simulink model "Citation"  (R2018a)
settings: Solver=ode5  StartTime=0.0  StopTime=500  FixedStep=0.01  RelTol=1e-3  EnableMultiTasking=on
InitFcn:
  | initcit
values from neighbouring files (symbols this model uses):
  aeroinit = [dp_ini;inicoef('CX0');inicoef('CXa');inicoef('CXa2');inicoef('CXq')     ;inicoef('CXde');inicoef('CY0');inicoef('CYB');inicoef('CYp');inicoef('CYr')     ;inicoef('CYda');inicoef('CYdr');inicoef('CZ0');inicoef('CZa');inicoef('CZq')     ;inicoef('CZde');inicoef('Cl0');inicoef('ClB');inicoef('Clp');inicoef('Clr')     ;inicoef('Clda');inicoef('Cldr');inicoef('Cm0');inicoef('Cma');inicoef('Cmq')     ; ...(+113 chars)    [initcit.m]
  h_l_old = zeros(6,sample_size)    [initcit.m]
  h_m_old = zeros(4,sample_size)    [initcit.m]
  h_n_old = zeros(6,sample_size)    [initcit.m]
  h_X_old = zeros(5,sample_size)    [initcit.m]
  h_Y_old = zeros(6,sample_size)    [initcit.m]
  h_Z_old = zeros(4,sample_size)    [initcit.m]
  I = [massinit(5),0, -massinit(8);0, massinit(6),0;-massinit(8),0, massinit(7)]    [initcit.m]
  p_l = [inicoef('Cl0');inicoef('ClB');inicoef('Clp');inicoef('Clr')     ;inicoef('Clda');inicoef('Cldr')].*ones(6,sample_size)    [initcit.m]
  p_m = [inicoef('Cm0');inicoef('Cma');inicoef('Cmq')     ;inicoef('Cmde')].*ones(4,sample_size)    [initcit.m]
  p_n = 0.71*ones(6,sample_size)    [initcit.m]
  p_X = [inicoef('CX0');inicoef('CXa');inicoef('CXa2');inicoef('CXq')     ;inicoef('CXde')].*ones(5,sample_size)    [initcit.m]
  p_Y = [inicoef('CY0');inicoef('CYB');inicoef('CYp');inicoef('CYr')     ;inicoef('CYda');inicoef('CYdr')].*ones(6,sample_size)    [initcit.m]
  p_Z = [inicoef('CZ0');inicoef('CZa');inicoef('CZq')     ;inicoef('CZde')].*ones(4,sample_size)    [initcit.m]
  Pcov_l = 10000*eye(6)    [initcit.m]
  Pcov_m = 10000*eye(4)    [initcit.m]
  Pcov_n = 10000*eye(6)    [initcit.m]
  Pcov_X = 10000*eye(5)    [initcit.m]
  Pcov_Y = 10000*eye(6)    [initcit.m]
  Pcov_Z = 10000*eye(4)    [initcit.m]
  T0 = 288.15    [rho_test.m]
  Vw915 = 0    [initcit.m]
  winddir = 45*(pi/180)    (= 0.785398163397)    [initcit.m]
  x0 = []    [cessnac550_3d_sfnc.m]    (also in sfunxyauto.m)
  y_l = zeros(1,sample_size)    [initcit.m]
  y_l_est_old = zeros(size(y_l))    [initcit.m]
  y_m = zeros(1,sample_size)    [initcit.m]
  y_m_est_old = zeros(size(y_m))    [initcit.m]
  y_n = zeros(1,sample_size)    [initcit.m]
  y_n_est_old = zeros(size(y_n))    [initcit.m]
  y_X = zeros(1,sample_size)    [initcit.m]
  y_X_est_old = zeros(size(y_X))    [initcit.m]
  y_Y = zeros(1,sample_size)    [initcit.m]
  y_Y_est_old = zeros(size(y_Y))    [initcit.m]
  y_Z = zeros(1,sample_size)    [initcit.m]
  y_Z_est_old = zeros(size(y_Z))    [initcit.m]
undefined symbols (not defined in the file or in its folder): chord, cv1, cv2, cv3, cv4, deltagmax1, deltagmax2, deltagmax3, deltagmax4, Deng, ealphag, ealphas, g0, hDME, hGS, kt1, kt2, kt3, lh, massinit, matbuaf, matdaf, matdam, matdbbf, matdeaf, matdgaf, matdqaf, matduaf, matdwaw, matedhr, mateif, matelhr, matemhr, matemv1, matemv2, matemve, matetam, mateuaf, matfaaf, matfaxl, matff, matibaf, matibb, matibmh, matipaf, matipmh, matiraf, matiuaf, matiwaf, matlaf, matlam, matleaf, matleam, matlgaf, matlqaf, matluaf, matmaaf, matmaam, matmaf, matmam ... (+75)
libraries: simulink x5, templibrary x3, vrlib x1
(part 1 of 6)
settings Model: ExtModeTrigMode=oneshot  ExtModeArmWhenConnect=off  Creator=laurensvaneykeren  LastModifiedBy=jelle
settings DataIOCC: SaveFormat=Array  SignalLoggingName=sigsOut
settings OptimizationCC: BooleanDataType=off  ExpressionDepthLimit=2147483647  LifeSpan=inf
settings DebuggingCC: SaveWithParameterizedLinksMsg=none  UnderspecifiedInitializationDetection=Classic  MergeDetectMultiDrivingBlocksExec=none  SignalResolutionControl=TryResolveAllWithWarning  MultiTaskDSMMsg=warning  MultiTaskCondExecSysMsg=none  FcnCallInpInsideContextMsg=warning  StateNameClashWarn=warning  SFUnexpectedBacktrackingDiag=warning  SFNoUnconditionalDefaultTransitionDiag=warning  SFExecutionAtInitializationDiag=none
settings HardwareCC: ProdBitPerPointer=32  ProdBitPerSizeT=32  ProdBitPerPtrDiffT=32  ProdLargestAtomicFloat=None  ProdIntDivRoundTo=Undefined  ProdEndianess=Unspecified  ProdWordSize=32  ProdHWDeviceType=32-bit Generic  TargetUnknown=on
settings ModelReferenceCC: PropagateSignalLabelsOutOfModel=off
settings RTWCC: SystemTargetFile=grt_malloc.tlc  GenCodeOnly=on  TemplateMakefile=grt_malloc_default_tmf
settings CodeAppCC: StateflowObjectComments=on
settings GRTTargetCC: TargetLangStandard=C89/C90 (ANSI)  CombineOutputUpdateFcns=off  GRTInterface=on  UseMalloc=on
settings ConfigComp: CovMetricSettings=dw  CovHtmlReporting=on  CovSaveCumulativeToWorkspaceVar=on  CovSaveSingleToWorkspaceVar=on  CovExternalEMLEnable=off

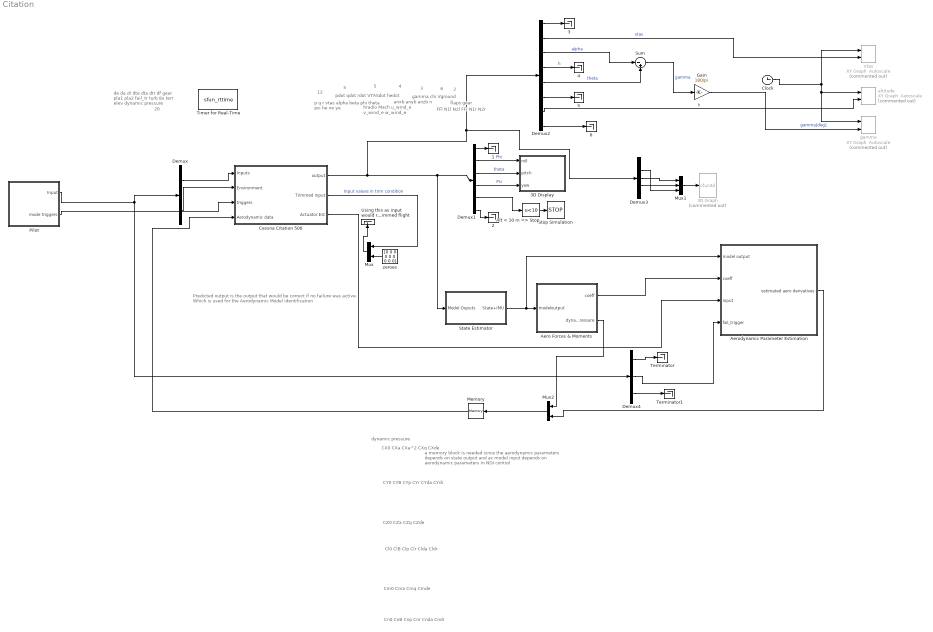
== system Citation ==
  note: a memory block is needed since the aerodynamic parameters depends on state output and ac model input depends on aerodynamic parameters in NDI control
  note: Predicted output is the output that would be correct if no failure was active.
      | Which is used for the Aerodynamic Model identification
  note: de
      | da
      | dr
      | dte
      | dta
      | dtr
      | df
      | gear
      | pla1
      | pla2
      | fail_tr
      | turb 8x
      | terr elev
      | dynamic pressure
  note: p
      | q
      | r
      | vtas
      | alpha
      | beta
      | phi
      | theta
      | psi
      | he
      | xe
      | ye
  note: pdot
      | qdot
      | rdot
      | VTASdot
      | hedot
  note: hradio
      | Mach
      | u_wind_e
      | v_wind_e
      | w_wind_e
  note: anxb
      | anyb
      | anzb
      | n
  note: gamma
      | chi
      | Vground
  note: flaps
      | gear
  note: FFl
      | N1l
      | N2l
      | FFr
      | N1r
      | N2r
  note: 12
  note: 5
  note: 5
  note: 4
  note: 3
  note: 6
  note: 2
  note: 20
  note: Cn0
      | CnB
      | Cnp
      | Cnr
      | Cnda
      | Cndr
  note: CZ0
      | CZa
      | CZq
      | CZde
  note: Cm0
      | Cma
      | Cmq
      | Cmde
  note: CY0
      | CYB
      | CYp
      | CYr
      | CYda
      | CYdr
  note: Cl0
      | ClB
      | Clp
      | Clr
      | Clda
      | Cldr
  note: CX0
      | CXa
      | CXa^2
      | CXq
      | CXde
  note: dynamic pressure
  {1..6} (6 alike) : Terminator
  3D Display : Subsystem
  3D Graph : S-Function  Commented=on  LoadFcn=if exist('sfun3d','file'), sfun3d([],[],[],'LoadBlock'); end  FunctionName=sfun3d  Parameters=ax,T,np,cp,gd,ls,mk,mx,hd,tb  SFunctionDeploymentMode=off  EnableBusSupport=off  mask(3D Graph){np=1, ax=[-5000 5000 -5000 5000 0 10000], mx=1e8, T=0.01, cp=[1 1 0.5], gd=on, hd=on, tb=on, ls=-, mk=none}
      mask prompts: np "Number of moving points (lines)"; ax "Range: [xmin xmax  ymin ymax zmin zmax]"; mx "Max number of points in each line"; T "Sampling Time"; cp "Camera position (use [0 0 1] for 2D XY view)"; gd "Grid (on|off)"; hd "HeadMarkers (on|off)"; tb "Toolbar (on|off)"; ls "LineStyle"; mk "LineMarker"
      mask help:
      | This block plots the position of several points in the XYZ space. The input contains the coordinates of all the points (x1,y1,z1,x2,y2,z2,...).
      | The number of moving points (lines), the XYZ ranges, sampling time, camera position, and grid (among other things) can be set as mask parameters.
      settings: CopyFcn=if exist('sfun3d','file'), sfun3d([],[],[],'CopyBlock'); end  DeleteFcn=if exist('sfun3d','file'), sfun3d([],[],[],'DeleteBlock'); end  NameChangeFcn=if exist('sfun3d','file'), sfun3d([],[],[],'NameChange'); end
      mask Help:
      | This block plots the position of several points in the XYZ space. The input contains the coordinates of all the points (x1,y1,z1,x2,y2,z2,...).
      | The number of moving points (lines), the XYZ ranges, sampling time, camera position, and grid (among other things) can be set as mask parameters.
      mask TypeOptions ls: - | -- | : | -. | none
      mask TypeOptions mk: none | . | + | o | * | x | square | diamond | v | ^ | > | < | pentagram | hexagram
      mask Display: plot([.05 .95 .95 .05 .05],[.45 .45 .95 .95 .45], 0.5+cos(0:0.1:2*pi)*0.3,0.7+sin(0:0.1:2*pi)*0.2)
  "Aero Forces & Moments " : Subsystem
  Aerodynamic Parameter Estimation : Subsystem
  Alt < 10 m => Stop : Fcn  Expr=u<10
  Cessna Citation 500 : Subsystem  mask(Citation Aircraft Model){trimdatafile=example.tri}
      mask prompts: trimdatafile "Trim Condition"
      mask init:
      | initcit;
      mask Display:
      | image(imread('Citation.jpg'))
      | port_label('input', 1, 'Inputs')
      | port_label('input', 2, 'Environment')
      | port_label('input', 4, 'Aerodynamic Data')
      | port_label('input', 3, 'Mode Triggers')
      | port_label('output', 1, 'Outputs')
      | port_label('output', 2, 'Trim inputs')
      | port_label('output', 3, 'Predicted Output')
  Clock : Clock
  Demux : Demux  Outputs=[11 9]
  Demux1 : Demux  Outputs=[6 1 1 1 1 27]
  Demux2 : Demux  Outputs=[3 1 1 2 1 1 1 27]
  Demux3 : Demux  Outputs=[9 1 1 1 25]
  Demux4 : Demux  Outputs=[10 1 9]
  Gain : Gain  Gain=180/pi
  Memory : Memory  InitialCondition=aeroinit
  Mux : Mux  Inputs=2
  Mux1 : Mux  Inputs=3
  Mux2 : Mux  Inputs=2
  Pilot : Subsystem
  "State Estimator " : Subsystem
  Stop Simulation : Stop
  Sum : Sum  Inputs=|-+
  Terminator : Terminator
  Terminator1 : Terminator
  Timer for Real-Time : S-Function  FunctionName=sfun_rttime  Parameters=1  SFunctionDeploymentMode=off  EnableBusSupport=off
  Using this as input would result in trimmed flight : Terminator
  Vtas : templibrary/XY Graph  Autoscale  Commented=on  xmin=-1  xmax=1  ymin=-1  ymax=1  st=0
  altitude : templibrary/XY Graph  Autoscale  Commented=on  xmin=-1  xmax=1  ymin=-1  ymax=1  st=0
      link override S-Function: Parameters="[xmin xmax ymin ymax],  st"
  gamma : templibrary/XY Graph  Autoscale  Commented=on  xmin=-1  xmax=1  ymin=-1  ymax=1  st=0
  zeroes : Constant  Value=[0 0 0 0 0 0 0 0 0]
  wires:
  Demux/1 -> Cessna Citation 500/1(Inputs)
  Pilot/1(Input) -> Demux/1, Demux4/1
  Cessna Citation 500/1(output) -> Demux3/1, Demux2/1, "State Estimator "/1(Model Ouputs), Demux1/1
  Demux/2 -> Cessna Citation 500/2(Environment)
  Cessna Citation 500/2(Trimmed input) -> Mux/1  "Input values in trim condition"
  zeroes/1 -> Mux/2
  Mux/1 -> Using this as input would result in trimmed flight/1
  Demux1/1 -> 1/1
  Demux1/5 -> Alt < 10 m => Stop/1
  Demux1/2 -> 3D Display/1(roll)  "Phi"
  Demux1/3 -> 3D Display/2(pitch)  "theta"
  Demux1/4 -> 3D Display/3(yaw)  "Psi"
  Alt < 10 m => Stop/1 -> Stop Simulation/1
  Demux1/6 -> 2/1
  "State Estimator "/1(State+IMU) -> Aerodynamic Parameter Estimation/1("model output "), "Aero Forces & Moments "/1(modeloutput)
  Cessna Citation 500/3(Actuator Est) -> Aerodynamic Parameter Estimation/3("input ")
  "Aero Forces & Moments "/1(coeff) -> Aerodynamic Parameter Estimation/2("coeff ")
  Demux2/1 -> 3/1
  Demux2/2 -> Vtas/2  "vtas"
  Demux2/3 -> Sum/1  "alpha"
  Demux2/4 -> 4/1  "h"
  Demux2/5 -> Sum/2  "theta"
  Demux2/7 -> altitude/2  "h"
  Demux2/6 -> 5/1
  Demux2/8 -> 6/1
  Sum/1 -> Gain/1  "gamma"
  Gain/1 -> gamma/2  "gamma[deg]"
  Demux3/2 -> Mux1/3
  Demux3/3 -> Mux1/1
  Demux3/4 -> Mux1/2
  Mux1/1 -> 3D Graph/1
  Clock/1 -> gamma/1, altitude/1, Vtas/1
  Demux4/2 -> Aerodynamic Parameter Estimation/4("fail_trigger ")
  Demux4/1 -> Terminator/1
  Demux4/3 -> Terminator1/1
  Aerodynamic Parameter Estimation/1(estimated aero derivatives) -> Mux2/2
  "Aero Forces & Moments "/2("dynamic pressure ") -> Mux2/1
  Mux2/1 -> Memory/1
  Memory/1 -> Cessna Citation 500/4("Aerodynamic data ")
  Pilot/2("mode triggers ") -> Cessna Citation 500/3(triggers)

== system Citation/3D Display ==
  roll : Inport
  pitch : Inport  Port=2
  yaw : Inport  Port=3
  Mux1 : Mux
  Position : Subsystem
  S-Function : S-Function  FunctionName=cessnac550_3d_sfnc  SFunctionDeploymentMode=off  EnableBusSupport=off
  Stop Simulation : Stop
  wires:
  roll/1 -> Mux1/1
  Position/1(Out1) -> Mux1/4
  pitch/1 -> Mux1/2
  yaw/1 -> Mux1/3
  Mux1/1 -> S-Function/1
  S-Function/1 -> Stop Simulation/1

== system Citation/Aero Forces & Moments  ==
  note: Kinematic Force Coeffient determination
  note: anxb
      | anyb
      | anzb
      | n
  note: hradio
      | Mach
      | u_wind_e
      | v_wind_e
      | w_wind_e
  note: p
      | q
      | r
      | vtas
      | alpha
      | beta
      | phi
      | theta
      | psi
      | he
      | xe
      | ye
  note: gamma
      | chi
      | Vground
  note: pdot
      | qdot
      | rdot
      | VTASdot
      | hedot
  note: FFl
      | N1l
      | N2l
      | FFr
      | N1r
      | N2r
  note: flaps
      | gear
  note: 6
  note: 5
  note: 12
  note: 3
  note: 5
  note: 4
  note: 2
  note: CX
      | CY
      | CZ
      | Cl
      | Cm
      | Cn
  modeloutput : Inport
  Aerodynamic Force Components : Subsystem
  Aerodynamic Moment Components : Subsystem
  Calculate Dynamic Pressure : Subsystem
  Mux : Mux  Inputs=2
  coeff : Outport
  "dynamic pressure " : Outport  Port=2
  wires:
  Aerodynamic Force Components/1(Out1) -> Mux/1
  modeloutput/1 -> Calculate Dynamic Pressure/1(In1), Aerodynamic Moment Components/1("State "), Aerodynamic Force Components/1("model output ")
  Calculate Dynamic Pressure/1(Out1) -> "dynamic pressure "/1, Aerodynamic Moment Components/2("Dynamic Pressure "), Aerodynamic Force Components/2(dynamic pressure)
  Aerodynamic Moment Components/1(Out1) -> Mux/2
  Mux/1 -> coeff/1

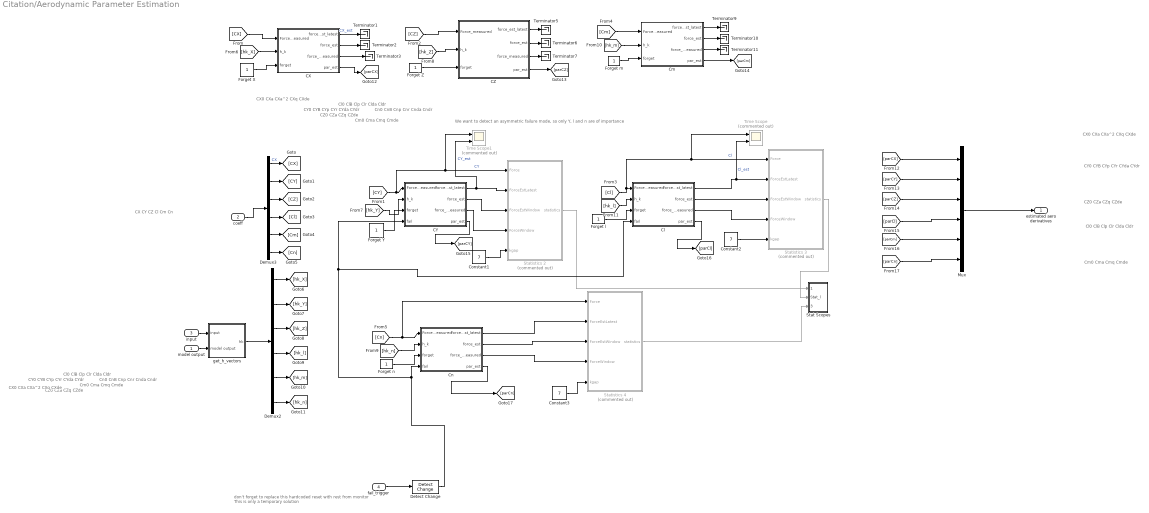
== system Citation/Aerodynamic Parameter Estimation ==
  note: don't forget to replace this hardcoded reset with rest from monitor
      | This is only a temporary solution
  note: We want to detect an asymmetric failure mode, so only Y, l and n are of importance
  note: CX
      | CY
      | CZ
      | Cl
      | Cm
      | Cn
  note: CX0
      | CXa
      | CXa^2
      | CXq
      | CXde
  note: CY0
      | CYB
      | CYp
      | CYr
      | CYda
      | CYdr
  note: CZ0
      | CZa
      | CZq
      | CZde
  note: Cl0
      | ClB
      | Clp
      | Clr
      | Clda
      | Cldr
  note: Cm0
      | Cma
      | Cmq
      | Cmde
  note: Cn0
      | CnB
      | Cnp
      | Cnr
      | Cnda
      | Cndr
  note: Cm0
      | Cma
      | Cmq
      | Cmde
  note: Cn0
      | CnB
      | Cnp
      | Cnr
      | Cnda
      | Cndr
  note: CY0
      | CYB
      | CYp
      | CYr
      | CYda
      | CYdr
  note: CZ0
      | CZa
      | CZq
      | CZde
  note: CX0
      | CXa
      | CXa^2
      | CXq
      | CXde
  note: Cl0
      | ClB
      | Clp
      | Clr
      | Clda
      | Cldr
  note: Cl0
      | ClB
      | Clp
      | Clr
      | Clda
      | Cldr
  note: CY0
      | CYB
      | CYp
      | CYr
      | CYda
      | CYdr
  note: Cm0
      | Cma
      | Cmq
      | Cmde
  note: CX0
      | CXa
      | CXa^2
      | CXq
      | CXde
  note: CZ0
      | CZa
      | CZq
      | CZde
  "model output " : Inport
  "coeff " : Inport  Port=2
  "input " : Inport  Port=3
  "fail_trigger " : Inport  Port=4
  CX : Subsystem
  CY : Subsystem
  CZ : Subsystem
  Cl : Subsystem
  Cm : Subsystem
  Cn : Subsystem
  Constant1 : Constant  Value=7
  Constant2 : Constant  Value=7
  Constant3 : Constant  Value=7
  Demux2 : Demux  Outputs=[5 6 4 6 4 6]
  Demux3 : Demux  Outputs=[1 1 1 1 1 1]
  Detect Change : simulink/Logic and Bit Operations/Detect Change  vinit=0  OutDataTypeStr=boolean
  Forget X : Constant
  Forget Y : Constant
  Forget Z : Constant
  Forget l : Constant
  Forget m : Constant
  Forget n : Constant
  Mux : Mux  Inputs=6
  "Stat Scopes " : Subsystem
  Statistics 2 : Subsystem  Commented=on
  Statistics 3 : Subsystem  Commented=on
  Statistics 4 : Subsystem  Commented=on
  Terminator{1..3,5..7,9..11} (9 alike) : Terminator
  Time Scope : Scope  Commented=on  NumInputPorts=2
  Time Scope1 : Scope  Commented=on  NumInputPorts=2
  get_h_vectors : Subsystem
  estimated aero derivatives : Outport
  wires:
  "input "/1 -> get_h_vectors/1(input)
  "model output "/1 -> get_h_vectors/2(model output)
  get_h_vectors/1(hk) -> Demux2/1
  "coeff "/1 -> Demux3/1
  Demux3/2 -> [CY]
  CX/4(par_est) -> [parCX]
  Forget X/1 -> CX/3(forget)
  Forget Y/1 -> CY/3(forget)
  Forget Z/1 -> CZ/3(forget)
  Forget l/1 -> Cl/3(forget)
  Forget m/1 -> Cm/3(forget)
  Forget n/1 -> Cn/3(forget)
  CY/1(force_est_latest) -> Time Scope1/2, Statistics 2/2(ForceEstLatest)  "CY_est"
  CY/2(force_est) -> Statistics 2/3(ForceEstWindow)
  CY/3(force_measured) -> Statistics 2/4(ForceWindow)
  Constant1/1 -> Statistics 2/5("kgap ")
  Cl/1(force_est_latest) -> Time Scope/2, Statistics 3/2(ForceEstLatest)  "Cl_est"
  Cl/2(force_est) -> Statistics 3/3(ForceEstWindow)
  Cl/3(force_measured) -> Statistics 3/4(ForceWindow)
  Constant2/1 -> Statistics 3/5("kgap ")
  Cn/1(force_est_latest) -> Statistics 4/2(ForceEstLatest)
  Cn/2(force_est) -> Statistics 4/3(ForceEstWindow)
  Constant3/1 -> Statistics 4/5("kgap ")
  Demux3/1 -> [CX]  "CX"
  [CX] -> CX/1(Force_measured)
  [CY] -> Time Scope1/1, Statistics 2/1(Force), CY/1(Force_measured)  "CY"
  Demux3/3 -> [CZ]
  [CZ] -> CZ/1(Force_measured)
  Demux3/4 -> [Cl]
  [Cl] -> Time Scope/1, Statistics 3/1(Force), Cl/1(Force_measured)  "Cl"
  Demux3/5 -> [Cm]
  [Cm] -> Cm/1(Force_measured)
  Demux3/6 -> [Cn]
  [Cn] -> Statistics 4/1(Force), Cn/1(Force_measured)
  Demux2/1 -> [hk_X]
  Demux2/2 -> [hk_Y]
  Demux2/3 -> [hk_Z]
  Demux2/4 -> [hk_l]
  Demux2/5 -> [hk_m]
  Demux2/6 -> [hk_n]
  [hk_X] -> CX/2(h_k)
  [hk_Y] -> CY/2(h_k)
  [hk_Z] -> CZ/2(h_k)
  [hk_l] -> Cl/2(h_k)
  [hk_m] -> Cm/2(h_k)
  [hk_n] -> Cn/2(h_k)
  Cn/3(force_measured) -> Statistics 4/4(ForceWindow)
  CX/1(force_est_latest) -> Terminator1/1  "CX_est"
  CX/2(force_est) -> Terminator2/1
  CX/3(force_measured) -> Terminator3/1
  CY/4(par_est) -> [parCY]
  CZ/2(force_est) -> Terminator6/1
  CZ/3(force_measured) -> Terminator7/1
  CZ/1(force_est_latest) -> Terminator5/1
  Cm/1(force_est_latest) -> Terminator9/1
  Cm/2(force_est) -> Terminator10/1
  Cm/3(force_measured) -> Terminator11/1
  Cm/4(par_est) -> [parCm]
  Statistics 4/1(statistics) -> "Stat Scopes "/3(Stat_n)
  Statistics 3/1(statistics) -> "Stat Scopes "/2(Stat_l)
  Statistics 2/1(statistics) -> "Stat Scopes "/1(Stat_Y)
  "fail_trigger "/1 -> Detect Change/1
  Detect Change/1 -> Cl/4("fail "), CY/4(fail), Cn/4("fail ")
  CZ/4(par_est) -> [parCZ]
  Cl/4(par_est) -> [parCl]
  Cn/4(par_est) -> [parCn]
  [parCX] -> Mux/1
  [parCY] -> Mux/2
  [parCZ] -> Mux/3
  [parCl] -> Mux/4
  [parCm] -> Mux/5
  [parCn] -> Mux/6
  Mux/1 -> estimated aero derivatives/1

== system Citation/Cessna Citation 500 ==
  note: output is actuator deflection before failure
  note: p
      | q
      | r
      | vtas
      | alpha
      | beta
      | phi
      | theta
      | psi
      | he
      | xe
      | ye
  note: de
      | da
      | dr
      | dte
      | dta
      | dtr
      | df
      | gear
      | pla1
      | pla2
  note: pdot
      | qdot
      | rdot
      | VTASdot
      | hedot
  note: hradio
      | Mach
      | u_wind_e
      | v_wind_e
      | w_wind_e
  note: anxb
      | anyb
      | anzb
      | n
  note: gamma
      | chi
      | Vground
  note: turb 8x
      | terr_elev
  note: flaps
      | gear
  note: de
      | da
      | dr
      | dte
      | dta
      | dtr
      | df
      | gear
      | pla1
      | pla2
  note: FFl
      | N1l
      | N2l
      | FFr
      | N1r
      | N2r
  note: fail_aileron
  Inputs : Inport
  Environment : Inport  Port=2
  triggers : Inport  Port=3
  "Aerodynamic data " : Inport  Port=4
  Actuators : Subsystem
  Citation model DASMAT : Subsystem
  Controllers : Subsystem
  Demux : Demux  Outputs=[10 1]
  Demux4 : Demux  Outputs=[8 2]
  Mux1 : Mux  Inputs=7
  Mux2 : Mux  Inputs=2
  trim conditions : Subsystem
  ua sel : Selector  IndexOptions=Index vector (dialog)  Indices=[5 6]  OutputSizes=1
  xdot sel : Selector  IndexOptions=Index vector (dialog)  Indices=[1 2 3 4 10]  OutputSizes=1
  yacc sel : Selector  IndexOptions=Index vector (dialog)  Indices=[4 5 6 15]  OutputSizes=1
  yair sel : Selector  IndexOptions=Index vector (dialog)  Indices=[6 9 22 23 24]  OutputSizes=1
  yfp sel : Selector  IndexOptions=Index vector (dialog)  Indices=[1 2 15]  OutputSizes=1
  ypp sel : Selector  IndexOptions=Index vector (dialog)  Indices=[2 3 4 13 14 15]  OutputSizes=1
  output : Outport
  Trimmed input : Outport  Port=2
  Actuator Est : Outport  Port=3
  wires:
  Mux1/1 -> output/1
  Citation model DASMAT/1(x) -> Mux1/1, Controllers/1(state)
  Demux4/1 -> Citation model DASMAT/1(ua), ua sel/1
  Demux4/2 -> Citation model DASMAT/2(ut)
  Citation model DASMAT/3(yair) -> yair sel/1
  yair sel/1 -> Mux1/3
  Citation model DASMAT/2(xdot) -> xdot sel/1
  xdot sel/1 -> Mux1/2
  yacc sel/1 -> Mux1/4
  Citation model DASMAT/4(yacc) -> yacc sel/1
  yfp sel/1 -> Mux1/5
  Citation model DASMAT/5(yfp) -> yfp sel/1
  Actuators/1(Actuator_True) -> Demux4/1
  trim conditions/1(ua) -> Mux2/1
  trim conditions/2(ut) -> Mux2/2
  Mux2/1 -> Trimmed input/1
  Controllers/1(control inputs) -> Actuators/1(In)
  ua sel/1 -> Mux1/7
  Citation model DASMAT/6(ypp) -> ypp sel/1
  ypp sel/1 -> Mux1/6
  Actuators/2(Actuator_est) -> Actuator Est/1
  Inputs/1 -> Demux/1
  Demux/1 -> Controllers/2(inputs)
  Demux/2 -> Actuators/2("failure trigger ")
  Environment/1 -> Citation model DASMAT/3(Environment)
  "Aerodynamic data "/1 -> Controllers/3(aerodata)
  triggers/1 -> Controllers/4("triggers ")

== system Citation/Pilot ==
  note: de
      | da
      | dr
      | dte
      | dta
      | dtr
      | df
      | gear
      | pla1
      | pla2
      | failure_tr
      | turb 8x
      | terr elev
  Joystick : Subsystem
  Mux : Mux  Inputs=13
  "button2toggle " : Subsystem
  button2toggle 1 : Subsystem
  da trim : Constant  Value=0
  de trim : Constant  Value=0
  delta flaps : Constant  Value=0
  dr trim : Constant  Value=0
  gear (ON=1/OFF=0) : Constant  Value=0
  terr elev : Constant  Value=0
  turb 8x : Constant  Value=zeros(1,8)
  Input : Outport
  "mode triggers " : Outport  Port=2
  wires:
  Mux/1 -> Input/1
  Joystick/1(delta elevator) -> Mux/1
  Joystick/3(delta rudder) -> Mux/3
  da trim/1 -> Mux/5
  de trim/1 -> Mux/4
  Joystick/2(delta aileron) -> Mux/2
  turb 8x/1 -> Mux/12
  terr elev/1 -> Mux/13
  Joystick/4(Throttle setting) -> Mux/10, Mux/9
  gear (ON=1/OFF=0)/1 -> Mux/8
  dr trim/1 -> Mux/6
  delta flaps/1 -> Mux/7
  Joystick/5("Failure Button ") -> "button2toggle "/1(In1)
  "button2toggle "/1(Out1) -> Mux/11
  Joystick/6(NDI Button) -> button2toggle 1/1(In1)
  button2toggle 1/1(Out1) -> "mode triggers "/1

== system Citation/State Estimator  ==
  note: It is assumed that the model ouputs are perfect measurements
  Model Ouputs : Inport
  State+IMU : Outport
  wires:
  Model Ouputs/1 -> State+IMU/1

== system Citation/3D Display/Position ==
  Mux2 : Mux  Inputs=3
  x : Constant  Value=0
  y : Constant  Value=0
  z : Constant  Value=0
  Out1 : Outport
  wires:
  y/1 -> Mux2/2
  z/1 -> Mux2/3
  x/1 -> Mux2/1
  Mux2/1 -> Out1/1

== system Citation/Aero Forces & Moments /Aerodynamic Force Components ==
  note: Massinit
      | [mass cg? ? ? Ixx Iyy Izz Ixz]
  note: State
  note: accelerations are given in [g]
  note: p
      | q
      | r
      | vtas
      | alpha
      | beta
      | phi
      | theta
      | psi
      | he
      | xe
      | ye
  note: gamma
      | chi
      | Vground
  note: hradio
      | Mach
      | u_wind_e
      | v_wind_e
      | w_wind_e
  note: anxb
      | anyb
      | anzb
      | n
  note: 5
  note: 12
  note: 4
  note: flaps
      | gear
  note: 3
  note: 6
  note: FFl
      | N1l
      | N2l
      | FFr
      | N1r
      | N2r
  note: 5
  note: pdot
      | qdot
      | rdot
      | VTASdot
      | hedot
  note: 2
  "model output " : Inport
  dynamic pressure : Inport  Port=2
  Constant : Constant  Value=massinit
  Demux : Demux  Outputs=[22 3 12]
  Demux2 : Demux  Outputs=[1 7]
  Divide : Product  Inputs=*/
  Gain : Gain  Gain=g0
  Product : Product
  Product2 : Product
  Terminator1 : Terminator
  Terminator2 : Terminator
  Terminator4 : Terminator
  Wing Area : Constant  Value=S
  Out1 : Outport
  wires:
  Demux/2 -> Gain/1
  Gain/1 -> Product2/1
  dynamic pressure/1 -> Product/1
  Wing Area/1 -> Product/2
  Product2/1 -> Divide/1
  Divide/1 -> Out1/1
  Product/1 -> Divide/2
  Demux/1 -> Terminator1/1
  Demux/3 -> Terminator2/1
  "model output "/1 -> Demux/1
  Demux2/1 -> Product2/2  "mass"
  Constant/1 -> Demux2/1
  Demux2/2 -> Terminator4/1

== system Citation/Aero Forces & Moments /Aerodynamic Moment Components ==
  note: p
      | q
      | r
      | vtas
      | alpha
      | beta
      | phi
      | theta
      | psi
      | he
      | xe
      | ye
  note: gamma
      | chi
      | Vground
  note: hradio
      | Mach
      | u_wind_e
      | v_wind_e
      | w_wind_e
  note: anxb
      | anyb
      | anzb
      | n
  note: 5
  note: 12
  note: 4
  note: flaps
      | gear
  note: 3
  note: 6
  note: FFl
      | N1l
      | N2l
      | FFr
      | N1r
      | N2r
  note: 5
  note: pdot
      | qdot
      | rdot
      | VTASdot
      | hedot
  note: 2
  note: Massinit
      | [mass cg? ? ? Ixx Iyy Izz Ixz]
  "State " : Inport
  "Dynamic Pressure " : Inport  Port=2
  Cl : Subsystem
  Cm : Subsystem
  Cn : Subsystem
  Mux : Mux  Inputs=3
  Out1 : Outport
  wires:
  "State "/1 -> Cl/1(model output), Cm/1("model output "), Cn/1(model output)
  "Dynamic Pressure "/1 -> Cn/2(Dynamic Pressure), Cm/2(Dynamic Pressure), Cl/2(Dynamic Pressure)
  Cl/1(Cl) -> Mux/1
  Cn/1(Cn) -> Mux/3
  Cm/1(Cm) -> Mux/2
  Mux/1 -> Out1/1

== system Citation/Aero Forces & Moments /Calculate Dynamic Pressure ==
  note: Dynamic Pressure
  In1 : Inport
  Calculate Air Density : MATLAB Function  TreatAsAtomicUnit=on
  Demux : Demux  Outputs=[3 1 33]
  Gain : Gain  Gain=0.5
  Product : Product
  Product1 : Product
  Terminator1 : Terminator
  Terminator2 : Terminator
  Out1 : Outport
  wires:
  Product/1 -> Product1/1  "V^2"
  Demux/3 -> Terminator2/1
  Demux/2 -> Product/2, Product/1  "Vtas"
  In1/1 -> Demux/1, Calculate Air Density/1(state)
  Product1/1 -> Gain/1
  Calculate Air Density/1(rho) -> Product1/2  "Rho"
  Demux/1 -> Terminator1/1
  Gain/1 -> Out1/1  "0.5*RHO*v^2"

== system Citation/Aerodynamic Parameter Estimation/CX ==
  note: counter is still obsolete
  note: if lambda=1 => no forgetting
  Force_measured : Inport
  h_k : Inport  Port=2
  forget : Inport  Port=3
  MATLAB Function : MATLAB Function  TreatAsAtomicUnit=on
  Memory1 : Memory
  Memory10 : Memory  InitialCondition=y_X
  Memory11 : Memory  InitialCondition=h_X_old
  Memory7 : Memory  InitialCondition=p_X
  Memory8 : Memory  InitialCondition=Pcov_X
  Memory9 : Memory  InitialCondition=y_X_est_old
  Selector : Selector  NumberOfDimensions=2  InputPortWidth=1  IndexOptions=Index vector (dialog),Index vector (dialog)  Indices=[1:5],1  OutputSizes=1,1
  Terminator : Terminator
  force_est_latest : Outport
  force_est : Outport  Port=2
  force_measured : Outport  Port=3
  par_est : Outport  Port=4
  wires:
  Memory9/1 -> MATLAB Function/6("y_est_old ")
  MATLAB Function/1(P_cov) -> Memory8/1
  Memory10/1 -> MATLAB Function/5("y_old ")
  MATLAB Function/5(h_old) -> Memory11/1
  Memory11/1 -> MATLAB Function/7("h_old ")
  MATLAB Function/3(y_old) -> Memory10/1, force_measured/1
  Memory7/1 -> MATLAB Function/2("pk ")
  MATLAB Function/4(y_est_old) -> Memory9/1, force_est/1
  Memory8/1 -> MATLAB Function/1("P_cov ")
  MATLAB Function/2(pk) -> Selector/1, Memory7/1
  h_k/1 -> MATLAB Function/4(hk_new)
  Force_measured/1 -> MATLAB Function/3("y_new ")
  MATLAB Function/6(counter) -> Memory1/1
  Memory1/1 -> MATLAB Function/8("counter ")
  forget/1 -> MATLAB Function/9(forget)  "lambda"
  MATLAB Function/7(y_est) -> force_est_latest/1
  MATLAB Function/8(y_new) -> Terminator/1  "y_new putthrough"
  Selector/1 -> par_est/1

== system Citation/Aerodynamic Parameter Estimation/CY ==
  note: reset covariance matrix to initial condition one time. whenever a failure has been detected
  note: if lambda=1 => no forgetting
  note: counter is still obsolete
  Force_measured : Inport
  h_k : Inport  Port=2
  forget : Inport  Port=3
  fail : Inport  Port=4
  Constant : Constant  Value=Pcov_Y
  MATLAB Function : MATLAB Function  TreatAsAtomicUnit=on
  Memory1 : Memory
  Memory10 : Memory  InitialCondition=y_Y
  Memory11 : Memory  InitialCondition=h_Y_old
  Memory7 : Memory  InitialCondition=p_Y
  Memory8 : Memory  InitialCondition=Pcov_Y
  Memory9 : Memory  InitialCondition=y_Y_est_old
  Selector : Selector  NumberOfDimensions=2  InputPortWidth=1  IndexOptions=Index vector (dialog),Index vector (dialog)  Indices=[1:6],1  OutputSizes=1,1
  Switch : Switch  Criteria=u2 > Threshold
  Terminator : Terminator
  force_est_latest : Outport
  force_est : Outport  Port=2
  force_measured : Outport  Port=3
  par_est : Outport  Port=4
  wires:
  MATLAB Function/8(y_new) -> Terminator/1  "y_new putthrough"
  MATLAB Function/7(y_est) -> force_est_latest/1
  forget/1 -> MATLAB Function/9(forget)  "lambda"
  Memory1/1 -> MATLAB Function/8("counter ")
  MATLAB Function/6(counter) -> Memory1/1
  Force_measured/1 -> MATLAB Function/3("y_new ")
  h_k/1 -> MATLAB Function/4(hk_new)
  MATLAB Function/2(pk) -> Selector/1, Memory7/1
  Memory8/1 -> Switch/3
  MATLAB Function/4(y_est_old) -> force_est/1, Memory9/1
  Memory7/1 -> MATLAB Function/2("pk ")
  MATLAB Function/3(y_old) -> force_measured/1, Memory10/1
  Memory11/1 -> MATLAB Function/7("h_old ")
  MATLAB Function/5(h_old) -> Memory11/1
  Memory10/1 -> MATLAB Function/5("y_old ")
  MATLAB Function/1(P_cov) -> Memory8/1
  Memory9/1 -> MATLAB Function/6("y_est_old ")
  fail/1 -> Switch/2
  Constant/1 -> Switch/1
  Switch/1 -> MATLAB Function/1("P_cov ")
  Selector/1 -> par_est/1

== system Citation/Aerodynamic Parameter Estimation/CZ ==
  note: counter is still obsolete
  note: if lambda=1 => no forgetting
  Force_measured : Inport
  h_k : Inport  Port=2
  forget : Inport  Port=3
  MATLAB Function : MATLAB Function  TreatAsAtomicUnit=on
  Memory1 : Memory
  Memory10 : Memory  InitialCondition=y_Z
  Memory11 : Memory  InitialCondition=h_Z_old
  Memory7 : Memory  InitialCondition=p_Z
  Memory8 : Memory  InitialCondition=Pcov_Z
  Memory9 : Memory  InitialCondition=y_Z_est_old
  Selector : Selector  NumberOfDimensions=2  InputPortWidth=1  IndexOptions=Index vector (dialog),Index vector (dialog)  Indices=[1:4],1  OutputSizes=1,1
  Terminator : Terminator
  force_est_latest : Outport
  force_est : Outport  Port=2
  force_measured : Outport  Port=3
  par_est : Outport  Port=4
  wires:
  Memory9/1 -> MATLAB Function/6("y_est_old ")
  MATLAB Function/1(P_cov) -> Memory8/1
  Memory10/1 -> MATLAB Function/5("y_old ")
  MATLAB Function/5(h_old) -> Memory11/1
  Memory11/1 -> MATLAB Function/7("h_old ")
  MATLAB Function/3(y_old) -> Memory10/1, force_measured/1
  Memory7/1 -> MATLAB Function/2("pk ")
  MATLAB Function/4(y_est_old) -> Memory9/1, force_est/1
  Memory8/1 -> MATLAB Function/1("P_cov ")
  MATLAB Function/2(pk) -> Memory7/1, Selector/1
  h_k/1 -> MATLAB Function/4(hk_new)
  Force_measured/1 -> MATLAB Function/3("y_new ")
  MATLAB Function/6(counter) -> Memory1/1
  Memory1/1 -> MATLAB Function/8("counter ")
  forget/1 -> MATLAB Function/9(forget)  "lambda"
  MATLAB Function/7(y_est) -> force_est_latest/1
  MATLAB Function/8(y_new) -> Terminator/1  "y_new putthrough"
  Selector/1 -> par_est/1

== system Citation/Aerodynamic Parameter Estimation/Cl ==
  note: if lambda=1 => no forgetting
  note: counter is still obsolete
  Force_measured : Inport
  h_k : Inport  Port=2
  forget : Inport  Port=3
  "fail " : Inport  Port=4
  Constant : Constant  Value=Pcov_l
  MATLAB Function : MATLAB Function  TreatAsAtomicUnit=on
  Memory1 : Memory
  Memory10 : Memory  InitialCondition=y_l
  Memory11 : Memory  InitialCondition=h_l_old
  Memory7 : Memory  InitialCondition=p_l
  Memory8 : Memory  InitialCondition=Pcov_l
  Memory9 : Memory  InitialCondition=y_l_est_old
  Selector : Selector  NumberOfDimensions=2  InputPortWidth=1  IndexOptions=Index vector (dialog),Index vector (dialog)  Indices=[1:6],1  OutputSizes=1,1
  Switch : Switch  Criteria=u2 > Threshold
  Terminator : Terminator
  force_est_latest : Outport
  force_est : Outport  Port=2
  force_measured : Outport  Port=3
  par_est : Outport  Port=4
  wires:
  MATLAB Function/8(y_new) -> Terminator/1  "y_new putthrough"
  MATLAB Function/7(y_est) -> force_est_latest/1
  forget/1 -> MATLAB Function/9(forget)  "lambda"
  Memory1/1 -> MATLAB Function/8("counter ")
  MATLAB Function/6(counter) -> Memory1/1
  Force_measured/1 -> MATLAB Function/3("y_new ")
  h_k/1 -> MATLAB Function/4(hk_new)
  MATLAB Function/2(pk) -> Selector/1, Memory7/1
  MATLAB Function/4(y_est_old) -> Memory9/1, force_est/1
  Memory7/1 -> MATLAB Function/2("pk ")
  MATLAB Function/3(y_old) -> force_measured/1, Memory10/1
  Memory11/1 -> MATLAB Function/7("h_old ")
  MATLAB Function/5(h_old) -> Memory11/1
  Memory10/1 -> MATLAB Function/5("y_old ")
  MATLAB Function/1(P_cov) -> Memory8/1
  Memory9/1 -> MATLAB Function/6("y_est_old ")
  "fail "/1 -> Switch/2
  Constant/1 -> Switch/1
  Memory8/1 -> Switch/3
  Switch/1 -> MATLAB Function/1("P_cov ")
  Selector/1 -> par_est/1

== system Citation/Aerodynamic Parameter Estimation/Cm ==
  note: counter is still obsolete
  note: if lambda=1 => no forgetting
  Force_measured : Inport
  h_k : Inport  Port=2
  forget : Inport  Port=3
  MATLAB Function : MATLAB Function  TreatAsAtomicUnit=on
  Memory1 : Memory
  Memory10 : Memory  InitialCondition=y_m
  Memory11 : Memory  InitialCondition=h_m_old
  Memory7 : Memory  InitialCondition=p_m
  Memory8 : Memory  InitialCondition=Pcov_m
  Memory9 : Memory  InitialCondition=y_m_est_old
  Selector : Selector  NumberOfDimensions=2  InputPortWidth=1  IndexOptions=Index vector (dialog),Index vector (dialog)  Indices=[1:4],1  OutputSizes=1,1
  Terminator : Terminator
  force_est_latest : Outport
  force_est : Outport  Port=2
  force_measured : Outport  Port=3
  par_est : Outport  Port=4
  wires:
  Memory9/1 -> MATLAB Function/6("y_est_old ")
  MATLAB Function/1(P_cov) -> Memory8/1
  Memory10/1 -> MATLAB Function/5("y_old ")
  MATLAB Function/5(h_old) -> Memory11/1
  Memory11/1 -> MATLAB Function/7("h_old ")
  MATLAB Function/3(y_old) -> Memory10/1, force_measured/1
  Memory7/1 -> MATLAB Function/2("pk ")
  MATLAB Function/4(y_est_old) -> Memory9/1, force_est/1
  Memory8/1 -> MATLAB Function/1("P_cov ")
  MATLAB Function/2(pk) -> Selector/1, Memory7/1
  h_k/1 -> MATLAB Function/4(hk_new)
  Force_measured/1 -> MATLAB Function/3("y_new ")
  MATLAB Function/6(counter) -> Memory1/1
  Memory1/1 -> MATLAB Function/8("counter ")
  forget/1 -> MATLAB Function/9(forget)  "lambda"
  MATLAB Function/7(y_est) -> force_est_latest/1
  MATLAB Function/8(y_new) -> Terminator/1  "y_new putthrough"
  Selector/1 -> par_est/1

== system Citation/Aerodynamic Parameter Estimation/Cn ==
  note: if lambda=1 => no forgetting
  note: counter is still obsolete
  Force_measured : Inport
  h_k : Inport  Port=2
  forget : Inport  Port=3
  "fail " : Inport  Port=4
  Constant : Constant  Value=Pcov_n
  MATLAB Function : MATLAB Function  TreatAsAtomicUnit=on
  Memory1 : Memory
  Memory10 : Memory  InitialCondition=y_n
  Memory11 : Memory  InitialCondition=h_n_old
  Memory7 : Memory  InitialCondition=p_n
  Memory8 : Memory  InitialCondition=Pcov_n
  Memory9 : Memory  InitialCondition=y_n_est_old
  Selector : Selector  NumberOfDimensions=2  InputPortWidth=1  IndexOptions=Index vector (dialog),Index vector (dialog)  Indices=[1:6],1  OutputSizes=1,1
  Switch : Switch  Criteria=u2 > Threshold
  Terminator : Terminator
  force_est_latest : Outport
  force_est : Outport  Port=2
  force_measured : Outport  Port=3
  par_est : Outport  Port=4
  wires:
  MATLAB Function/8(y_new) -> Terminator/1  "y_new putthrough"
  MATLAB Function/7(y_est) -> force_est_latest/1
  forget/1 -> MATLAB Function/9(forget)  "lambda"
  Memory1/1 -> MATLAB Function/8("counter ")
  MATLAB Function/6(counter) -> Memory1/1
  Force_measured/1 -> MATLAB Function/3("y_new ")
  h_k/1 -> MATLAB Function/4(hk_new)
  MATLAB Function/2(pk) -> Selector/1, Memory7/1
  MATLAB Function/4(y_est_old) -> force_est/1, Memory9/1
  Memory7/1 -> MATLAB Function/2("pk ")
  MATLAB Function/3(y_old) -> force_measured/1, Memory10/1
  Memory11/1 -> MATLAB Function/7("h_old ")
  MATLAB Function/5(h_old) -> Memory11/1
  Memory10/1 -> MATLAB Function/5("y_old ")
  MATLAB Function/1(P_cov) -> Memory8/1
  Memory9/1 -> MATLAB Function/6("y_est_old ")
  "fail "/1 -> Switch/2
  Constant/1 -> Switch/1
  Memory8/1 -> Switch/3
  Switch/1 -> MATLAB Function/1("P_cov ")
  Selector/1 -> par_est/1

== system Citation/Aerodynamic Parameter Estimation/Stat Scopes  ==
  note: variance
      | sigma_avg
      | sigma_avg
      | moving average
      | AutoCorr
      | AutoCorr_avg
  Stat_Y : Inport
  Stat_l : Inport  Port=2
  Stat_n : Inport  Port=3
  Demux : Demux  Outputs=6
  Demux1 : Demux  Outputs=6
  Demux4 : Demux  Outputs=6
  "Y Auto Correlation " : Scope  Commented=on  NumInputPorts=2
  Y moving average : Scope  Commented=on
  Y variance : Scope  Commented=on  NumInputPorts=3
  wires:
  Stat_l/1 -> Demux/1
  Demux/2 -> ?
  Demux1/4 -> Y moving average/1
  Demux4/2 -> ?
  Stat_Y/1 -> Demux1/1
  Demux/4 -> ?
  Stat_n/1 -> Demux4/1
  Demux4/1 -> ?
  Demux/1 -> ?
  Demux4/4 -> ?
  Demux/3 -> ?
  Demux4/3 -> ?
  Demux1/1 -> Y variance/1
  Demux1/2 -> Y variance/2
  Demux1/3 -> Y variance/3
  Demux1/5 -> "Y Auto Correlation "/1  "AutoCorr"
  Demux1/6 -> "Y Auto Correlation "/2  "AutoCorr avg"

== system Citation/Aerodynamic Parameter Estimation/Statistics 2 ==
  note: variance
      | sigma_avg
      | sigma_avg
      | moving average
      | AutoCorr
      | AutoCorr_avg
  Force : Inport
  ForceEstLatest : Inport  Port=2
  ForceEstWindow : Inport  Port=3
  ForceWindow : Inport  Port=4
  "kgap " : Inport  Port=5
  Auto_correlation : Subsystem
  Floor : Rounding
  Mux : Mux  Inputs=5
  Sum : Sum  Inputs=|-+
  Sum1 : Sum  Inputs=|+-
  moving average square : MATLAB Function  TreatAsAtomicUnit=on
  variance : Subsystem
  statistics : Outport
  wires:
  Sum/1 -> Auto_correlation/1(delta_window), moving average square/1(delta)
  Sum1/1 -> variance/1(delta)  "delta"
  "kgap "/1 -> Floor/1
  Floor/1 -> Auto_correlation/2(kgap)
  ForceWindow/1 -> Sum/2
  ForceEstWindow/1 -> Sum/1
  ForceEstLatest/1 -> Sum1/2
  Force/1 -> Sum1/1
  variance/1(variance) -> Mux/1
  variance/2(sigma_avg) -> Mux/2
  moving average square/1(av) -> Mux/3
  Auto_correlation/1(PI_kgap) -> Mux/4
  Auto_correlation/2(PI_kgap_avg) -> Mux/5
  Mux/1 -> statistics/1

== system Citation/Aerodynamic Parameter Estimation/Statistics 3 ==
  note: variance
      | sigma_avg
      | sigma_avg
      | moving average
      | AutoCorr
      | AutoCorr_avg
  Force : Inport
  ForceEstLatest : Inport  Port=2
  ForceEstWindow : Inport  Port=3
  ForceWindow : Inport  Port=4
  "kgap " : Inport  Port=5
  Auto_correlation : Subsystem
  Floor : Rounding
  Mux : Mux  Inputs=5
  Sum : Sum  Inputs=|-+
  Sum1 : Sum  Inputs=|+-
  moving average square : MATLAB Function  TreatAsAtomicUnit=on
  variance : Subsystem
  statistics : Outport
  wires:
  Mux/1 -> statistics/1
  Auto_correlation/2(PI_kgap_avg) -> Mux/5
  Auto_correlation/1(PI_kgap) -> Mux/4
  moving average square/1(av) -> Mux/3
  variance/2(sigma_avg) -> Mux/2
  variance/1(variance) -> Mux/1
  Force/1 -> Sum1/1
  ForceEstLatest/1 -> Sum1/2
  ForceEstWindow/1 -> Sum/1
  ForceWindow/1 -> Sum/2
  Floor/1 -> Auto_correlation/2(kgap)
  "kgap "/1 -> Floor/1
  Sum1/1 -> variance/1(delta)  "delta"
  Sum/1 -> moving average square/1(delta), Auto_correlation/1(delta_window)

== system Citation/Aerodynamic Parameter Estimation/Statistics 4 ==
  note: variance
      | sigma_avg
      | sigma_avg
      | moving average
      | AutoCorr
      | AutoCorr_avg
  Force : Inport
  ForceEstLatest : Inport  Port=2
  ForceEstWindow : Inport  Port=3
  ForceWindow : Inport  Port=4
  "kgap " : Inport  Port=5
  Auto_correlation : Subsystem
  Floor : Rounding
  Mux : Mux  Inputs=5
  Sum : Sum  Inputs=|-+
  Sum1 : Sum  Inputs=|+-
  moving average square : MATLAB Function  TreatAsAtomicUnit=on
  variance : Subsystem
  statistics : Outport
  wires:
  Sum/1 -> Auto_correlation/1(delta_window), moving average square/1(delta)
  Sum1/1 -> variance/1(delta)  "delta"
  "kgap "/1 -> Floor/1
  Floor/1 -> Auto_correlation/2(kgap)
  ForceWindow/1 -> Sum/2
  ForceEstWindow/1 -> Sum/1
  ForceEstLatest/1 -> Sum1/2
  Force/1 -> Sum1/1
  variance/1(variance) -> Mux/1
  variance/2(sigma_avg) -> Mux/2
  moving average square/1(av) -> Mux/3
  Auto_correlation/1(PI_kgap) -> Mux/4
  Auto_correlation/2(PI_kgap_avg) -> Mux/5
  Mux/1 -> statistics/1

== system Citation/Aerodynamic Parameter Estimation/get_h_vectors ==
  input : Inport
  model output : Inport  Port=2
  1 : Terminator
  6 : Terminator
  Constant : Constant
  Constant1 : Constant  Value=chord
  Constant2 : Constant  Value=span
  Demux4 : Demux  Outputs=[1 1 1 1 1 1 31]
  Demux5 : Demux  Outputs=[1 1 1 7]
  Divide : Product  Inputs=*/
  Divide1 : Product  Inputs=*/
  Divide2 : Product  Inputs=*/
  Gain : Gain  Gain=2
  Multiply : Product
  Multiply1 : Product
  Mux : Mux  Inputs=6
  Mux1 : Mux  Inputs=5
  Mux2 : Mux
  Mux3 : Mux  Inputs=6
  Product : Product
  Product1 : Product
  hk : Outport
  wires:
  Demux5/2 -> Mux/5  "da"
  Demux4/6 -> Mux/2  "beta"
  Demux4/5 -> Mux1/2, Product/2, Mux2/2, Product/1  "alpha"
  Constant/1 -> Mux1/1, Mux/1, Mux2/1
  Demux4/3 -> Multiply1/1  "r"
  Demux5/4 -> 6/1
  Demux4/2 -> Product1/1  "q"
  Demux4/1 -> Multiply/2  "p"
  Demux4/4 -> Gain/1, Divide/2  "vtas"
  Constant1/1 -> Product1/2
  Product1/1 -> Divide/1
  Divide/1 -> Mux2/3, Mux1/4  "qc/V"
  model output/1 -> Demux4/1
  Demux5/1 -> Mux2/4, Mux1/5  "de"
  Product/1 -> Mux1/3
  Demux5/3 -> Mux/6  "dr"
  input/1 -> Demux5/1
  Mux1/1 -> Mux3/1  "hk_CX"
  Mux2/1 -> Mux3/3, Mux3/5  "hk_CZ & hk_Cm"
  Demux4/7 -> 1/1
  Constant2/1 -> Multiply1/2, Multiply/1
  Multiply/1 -> Divide1/1
  Gain/1 -> Divide2/2, Divide1/2
  Divide1/1 -> Mux/3  "pb/2V"
  Multiply1/1 -> Divide2/1
  Divide2/1 -> Mux/4  "rb/2V"
  Mux/1 -> Mux3/2, Mux3/6, Mux3/4
  Mux3/1 -> hk/1

== system Citation/Cessna Citation 500/Actuators ==
  note: Failure will not be visible here
  note: de
      | da
      | dr
      | dte
      | dta
      | dtr
      | df
      | gear
      | pla1
      | pla2
  note: de
      | da
      | dr
      | dte
      | dta
      | dtr
      | df
      | gear
      | pla1
      | pla2
  In : Inport
  "failure trigger " : Inport  Port=2
  Demux : Demux  Outputs=10
  Gain : Gain  Gain=0.5
  Mux : Mux  Inputs=10
  Mux2 : Mux  Inputs=10
  Sum : Sum  Inputs=|++
  Switch : Switch  Criteria=u2 > Threshold
  "aileron failure offset (deg) " : Constant  Value=16
  da : Subsystem
  da limits : Saturate  UpperLimit=0.65  LowerLimit=-0.65
  de : Subsystem
  de limits : Saturate  UpperLimit=0.26  LowerLimit=-0.35
  deg2rad : Gain  Gain=pi/180
  dr : Subsystem
  dr limits : Saturate  UpperLimit=0.38  LowerLimit=-0.38
  flaps : Subsystem
  gear : Subsystem
  Actuator_True : Outport
  Actuator_est : Outport  Port=2
  wires:
  In/1 -> Demux/1
  Mux/1 -> Actuator_True/1
  Demux/1 -> de/1(In)
  Demux/2 -> da/1(In)
  Demux/3 -> dr/1(In)
  de/1(Out) -> de limits/1
  da/1(Out) -> da limits/1
  dr/1(Out) -> dr limits/1
  dr limits/1 -> Mux2/3, Mux/3
  de limits/1 -> Mux/1, Mux2/1
  Demux/8 -> gear/1(In)
  Demux/7 -> flaps/1(In)
  Demux/9 -> Mux2/9, Mux/9
  Demux/10 -> Mux2/10, Mux/10
  flaps/1(Out) -> Mux2/7, Mux/7
  gear/1(Out) -> Mux/8, Mux2/8
  Demux/4 -> Mux2/4, Mux/4
  Demux/5 -> Mux2/5, Mux/5
  Demux/6 -> Mux2/6, Mux/6
  da limits/1 -> Mux2/2, Switch/3, Gain/1
  "failure trigger "/1 -> Switch/2
  "aileron failure offset (deg) "/1 -> deg2rad/1
  deg2rad/1 -> Sum/1
  Gain/1 -> Sum/2
  Sum/1 -> Switch/1
  Switch/1 -> Mux/2
  Mux2/1 -> Actuator_est/1

== system Citation/Cessna Citation 500/Citation model DASMAT ==
  ua : Inport
  ut : Inport  Port=2
  Environment : Inport  Port=3
  AIRCRAFT MODEL : Subsystem
  Mux1 : Mux  Inputs=[8 2 8 12 8]
  Terminator_{16..19} (4 alike) : Terminator
  massinit : Constant  Value=massinit
  x : Outport
  xdot : Outport  Port=2
  yair : Outport  Port=3
  yacc : Outport  Port=4
  yfp : Outport  Port=5
  ypp : Outport  Port=6
  wires:
  AIRCRAFT MODEL/13(FMt) -> Terminator_19/1
  Mux1/1 -> yair/1
  AIRCRAFT MODEL/12(FMag) -> Terminator_17/1
  AIRCRAFT MODEL/11(FMa) -> Terminator_18/1
  AIRCRAFT MODEL/7(gust) -> Mux1/5
  AIRCRAFT MODEL/6(wind) -> Mux1/4
  AIRCRAFT MODEL/5(yad2) -> Mux1/3
  AIRCRAFT MODEL/4(yad1) -> Mux1/2
  AIRCRAFT MODEL/3(yatm) -> Mux1/1
  AIRCRAFT MODEL/2(xdot) -> xdot/1
  AIRCRAFT MODEL/1(x) -> x/1
  AIRCRAFT MODEL/10(ys) -> Terminator_16/1
  AIRCRAFT MODEL/9(yfp) -> yfp/1
  AIRCRAFT MODEL/8(yacc) -> yacc/1
  massinit/1 -> AIRCRAFT MODEL/3(massinit)
  ut/1 -> AIRCRAFT MODEL/2(ut)
  ua/1 -> AIRCRAFT MODEL/1(ua)
  Environment/1 -> AIRCRAFT MODEL/4(Environment)
  AIRCRAFT MODEL/14(ypp) -> ypp/1

== system Citation/Cessna Citation 500/Controllers ==
  note: Aerodata Description
  note: [1]
  note: p
      | q
      | r
      | vtas
      | alpha
      | beta
      | phi
      | theta
      | psi
      | he
      | xe
      | ye
  note: de
      | da
      | dr
      | dte
      | dta
      | dtr
      | df
      | gear
      | pla1
      | pla2
  note: CX0
      | CXa
      | CXa^2
      | CXq
      | CXde
  note: Cm0
      | Cma
      | Cmq
      | Cmde
  note: CY0
      | CYB
      | CYp
      | CYr
      | CYda
      | CYdr
  note: CZ0
      | CZa
      | CZq
      | CZde
  note: Cn0
      | CnB
      | Cnp
      | Cnr
      | Cnda
      | Cndr
  note: dynamic pressure
  note: Cl0
      | ClB
      | Clp
      | Clr
      | Clda
      | Cldr
  note: [2:6]
  note: [7:12]
  note: [13:16]
  note: [17:22]
  note: [23:26]
  note: [27:32]
  state : Inport
  inputs : Inport  Port=2
  aerodata : Inport  Port=3
  "triggers " : Inport  Port=4
  A/T disabled : Gain  SaturateOnIntegerOverflow=on  OutDataTypeStr=Inherit: Same as input  ParamDataTypeStr=Inherit: Same as input
  Display : Display
  Gain : Gain  Gain=0
  NDI Switch1 : ManualSwitch  Commented=on
  NDI rotational rate controller : Subsystem
  Switch : Switch  Criteria=u2 > Threshold
  Yaw damper : Subsystem
  add controller outputs to pilot inputs : Sum  Inputs=|+|+|+|  SaturateOnIntegerOverflow=on
  auto throttle : Subsystem
  beta feedback : Subsystem
  control inputs : Outport
  wires:
  state/1 -> NDI rotational rate controller/2(A/C state), beta feedback/1(state), Yaw damper/1(state), auto throttle/1(state)
  inputs/1 -> Switch/3, NDI rotational rate controller/1(inputs)
  add controller outputs to pilot inputs/1 -> control inputs/1
  auto throttle/1(controller output) -> A/T disabled/1
  A/T disabled/1 -> add controller outputs to pilot inputs/2
  Yaw damper/1(controller output) -> Gain/1
  Gain/1 -> add controller outputs to pilot inputs/1
  Switch/1 -> auto throttle/2(inputs), Yaw damper/2(inputs), beta feedback/2(input), add controller outputs to pilot inputs/3
  aerodata/1 -> NDI rotational rate controller/3(aero data)
  "triggers "/1 -> Display/1, Switch/2
  NDI rotational rate controller/1(control input) -> Switch/1

== system Citation/Cessna Citation 500/trim conditions ==
  PLA1/Tx1 : Constant  Value=ut0(1)
  PLA2/Tx2 : Constant  Value=ut0(2)
  control inputs : Mux  Inputs=8
      settings: DisplayOption=signals
  deltaa : Constant  Value=u0(2)
  deltae : Constant  Value=u0(1)
  deltaf : Constant  Value=u0(7)
  deltar : Constant  Value=u0(3)
  deltata : Constant  Value=u0(5)
  deltate : Constant  Value=u0(4)
  deltatr : Constant  Value=u0(6)
  engine inputs : Mux  Inputs=2
      settings: DisplayOption=signals
  lgsw : Constant  Value=u0(8)
  ua : Outport
  ut : Outport  Port=2
  wires:
  deltaf/1 -> control inputs/7  "df"
  engine inputs/1 -> ut/1
  deltatr/1 -> control inputs/6  "dtr"
  deltata/1 -> control inputs/5  "dta"
  control inputs/1 -> ua/1
  PLA1/Tx1/1 -> engine inputs/1  "pla1"
  PLA2/Tx2/1 -> engine inputs/2  "pla2"
  deltae/1 -> control inputs/1  "de"
  deltaa/1 -> control inputs/2  "da"
  deltar/1 -> control inputs/3  "dr"
  deltate/1 -> control inputs/4  "dte"
  lgsw/1 -> control inputs/8  "lg"

== system Citation/Pilot/Joystick ==
  note: Set to correct ID when switching between joysticks
  Demux : Demux  Outputs=6
  DualShock : Subsystem  Commented=on
  Joystick Input : vrlib/Joystick Input  joyid=1  adjustports=on  forcefeed=off
      settings: SourceProductBaseCode=VR
  Logitech 3D Pro : Subsystem
  Mux : Mux  Inputs=2
  Sum : Sum  Inputs=|++
  Terminator5 : Terminator
  delta elevator : Outport
  delta aileron : Outport  Port=2
  delta rudder : Outport  Port=3
  Throttle setting : Outport  Port=4
  "Failure Button " : Outport  Port=5
  NDI Button : Outport  Port=6
  wires:
  Joystick Input/3 -> Terminator5/1
  Joystick Input/1 -> Mux/1
  Joystick Input/2 -> Mux/2
  DualShock/1("Model Input ") -> Sum/1
  Logitech 3D Pro/1(Model Input) -> Sum/2
  Sum/1 -> Demux/1
  Demux/1 -> delta aileron/1
  Demux/2 -> delta elevator/1
  Demux/3 -> Throttle setting/1
  Demux/4 -> delta rudder/1
  Demux/5 -> "Failure Button "/1
  Mux/1 -> Logitech 3D Pro/1("JoyStick Input ")
  Demux/6 -> NDI Button/1

== system Citation/Pilot/button2toggle  ==
  In1 : Inport
  Constant1 : Constant
  Constant2 : Constant  Value=0
  Memory : Memory
  Switch : Switch  Criteria=u2 > Threshold
  Triggered Subsystem : Subsystem  TreatAsAtomicUnit=on
  Out1 : Outport
  wires:
  Memory/1 -> Switch/2
  Switch/1 -> Triggered Subsystem/1(In1)
  Constant2/1 -> Switch/1
  In1/1 -> Triggered Subsystem/Trigger
  Constant1/1 -> Switch/3
  Triggered Subsystem/1(Out1) -> Out1/1, Memory/1

== system Citation/Pilot/button2toggle 1 ==
  In1 : Inport
  Constant1 : Constant
  Constant2 : Constant  Value=0
  Memory : Memory
  Switch : Switch  Criteria=u2 > Threshold
  Triggered Subsystem : Subsystem  TreatAsAtomicUnit=on
  Out1 : Outport
  wires:
  Triggered Subsystem/1(Out1) -> Memory/1, Out1/1
  Constant1/1 -> Switch/3
  In1/1 -> Triggered Subsystem/Trigger
  Constant2/1 -> Switch/1
  Switch/1 -> Triggered Subsystem/1(In1)
  Memory/1 -> Switch/2

== system Citation/Aero Forces & Moments /Aerodynamic Moment Components/Cl ==
  note: (q*r*(Izz-Iyy)*)+(pdot*Ixx)-(Ixz*(pq+rdot))
  model output : Inport
  Dynamic Pressure : Inport  Port=2
  Constant : Constant  Value=S
  Constant1 : Constant  Value=span
  Demux : Demux  Outputs=[1 1 1 9 1 1 1 22]
  Demux1 : Demux  Outputs=[4 1 1 1 1]
  Divide : Product  Inputs=*/
  "Ixz*(pq+rdot) " : Product
  Product : Product  Inputs=3
  Sum : Sum  Inputs=|-+
  Sum1 : Sum  Inputs=|++
  Sum2 : Sum  Inputs=|-++
  Terminator{,1..2,6} (4 alike) : Terminator
  massinit : Constant  Value=massinit
  "pdot*Ixx " : Product
  pq : Product
  q*r*(Izz-Iyy) : Product  Inputs=3
  Cl : Outport
  wires:
  Demux/4 -> Terminator/1
  Demux/2 -> q*r*(Izz-Iyy)/1, pq/2  "q"
  Demux/5 -> "pdot*Ixx "/1  "pdot"
  massinit/1 -> Demux1/1
  Demux/1 -> pq/1  "p"
  Demux/8 -> Terminator1/1
  Demux1/2 -> "pdot*Ixx "/2  "Ixx"
  Demux/6 -> Terminator6/1  "qdot"
  Demux1/1 -> Terminator2/1
  model output/1 -> Demux/1
  Demux1/5 -> "Ixz*(pq+rdot) "/2  "Ixz"
  Demux/7 -> Sum1/2  "rdot"
  Demux/3 -> q*r*(Izz-Iyy)/2  "r"
  Demux1/3 -> Sum/1  "Iyy"
  Demux1/4 -> Sum/2  "Izz"
  Sum/1 -> q*r*(Izz-Iyy)/3
  pq/1 -> Sum1/1
  Sum1/1 -> "Ixz*(pq+rdot) "/1
  "Ixz*(pq+rdot) "/1 -> Sum2/1
  q*r*(Izz-Iyy)/1 -> Sum2/2
  "pdot*Ixx "/1 -> Sum2/3
  Dynamic Pressure/1 -> Product/1
  Constant/1 -> Product/2
  Constant1/1 -> Product/3
  Sum2/1 -> Divide/1
  Product/1 -> Divide/2
  Divide/1 -> Cl/1
